simulink model "Lecture2_Exercise_Sim"  (R2023b)
settings: Solver=VariableStepAuto  StartTime=0.0  StopTime=5  RelTol=1e-3
values from neighbouring files (symbols this model uses):
  Bm = 5 * 10^(-3)    (= 0.005)    [Lab_Assignment_5XWB0.m]
  Jm = 16.9 * 10^(-3)    (= 0.0169)    [Lab_Assignment_5XWB0.m]
  Kb = 1.01    [Lab_Assignment_5XWB0.m]
  La = 10.8 * 10^(-3)    (= 0.0108)    [Lab_Assignment_5XWB0.m]
  Lf = 58.4    [Lab_Assignment_5XWB0.m]
  Ra = 1.93    [Lab_Assignment_5XWB0.m]
  Rf = 276    [Lab_Assignment_5XWB0.m]
  Tl = 5    [Lab_Assignment_5XWB0.m]
  Vfmax = 310    [Lab_Assignment_5XWB0.m]
settings Model: Creator=20210999  LastModifiedBy=20210999

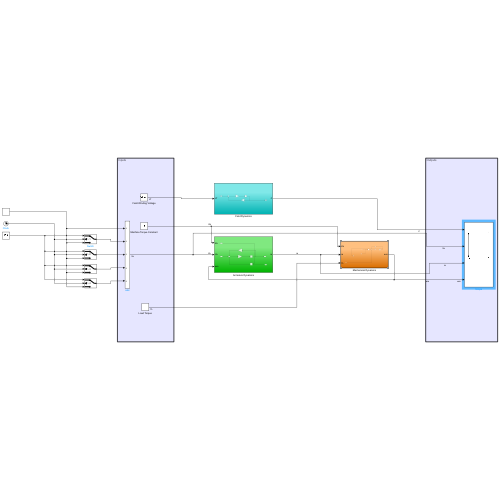
[thumbnail: Simulink's stored preview of the top-level diagram]
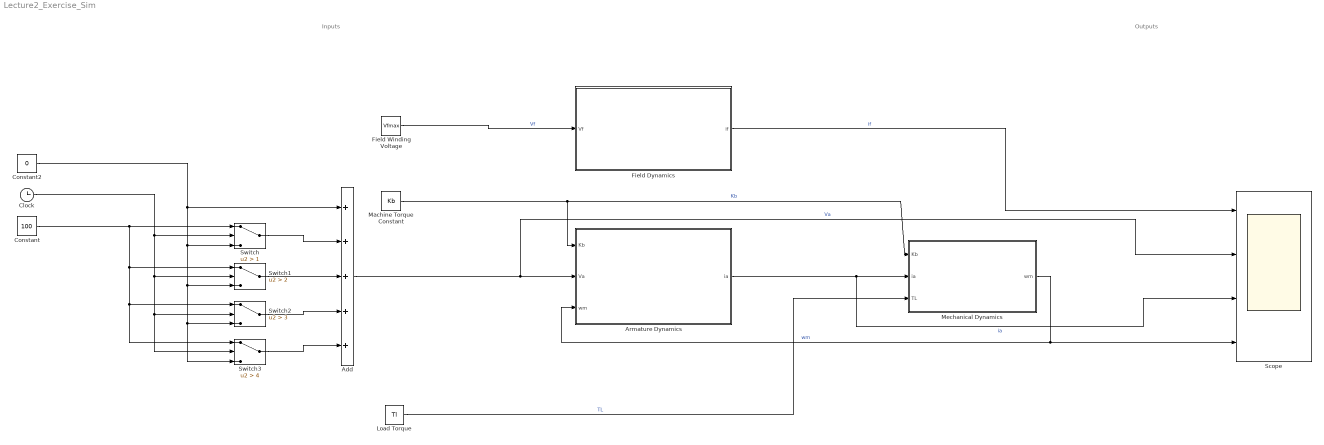
== system Lecture2_Exercise_Sim ==
  note: Inputs
  note: Outputs
  Add : Sum  Inputs=+++++
  Armature Dynamics : Subsystem
  Clock : Clock
      settings: Decimation=5
  Constant : Constant  Value=100
  Constant2 : Constant  Value=0
  Field Dynamics : Subsystem
  Field Winding Voltage : Constant  Value=Vfmax
  Load Torque : Constant  Value=Tl
  Machine Torque Constant : Constant  Value=Kb
  Mechanical Dynamics : Subsystem
  Scope : Scope  NumInputPorts=4
  Switch : Switch  Criteria=u2 > Threshold  Threshold=1  SaturateOnIntegerOverflow=off  InputSameDT=off
  Switch1 : Switch  Criteria=u2 > Threshold  Threshold=2  SaturateOnIntegerOverflow=off  InputSameDT=off
  Switch2 : Switch  Criteria=u2 > Threshold  Threshold=3  SaturateOnIntegerOverflow=off  InputSameDT=off
  Switch3 : Switch  Criteria=u2 > Threshold  Threshold=4  SaturateOnIntegerOverflow=off  InputSameDT=off
  wires:
  Field Winding Voltage/1 -> Field Dynamics/1(Vf)  "Vf"
  Machine Torque Constant/1 -> Armature Dynamics/1(Kb), Mechanical Dynamics/1(Kb)  "Kb"
  Armature Dynamics/1(ia) -> Scope/3, Mechanical Dynamics/2(ia)  "ia"
  Load Torque/1 -> Mechanical Dynamics/3(TL)  "TL"
  Mechanical Dynamics/1(wm) -> Scope/4, Armature Dynamics/3(wm)  "wm"
  Field Dynamics/1(if) -> Scope/1  "if"
  Clock/1 -> Switch3/2, Switch2/2, Switch1/2, Switch/2
  Constant2/1 -> Switch3/3, Switch2/3, Switch1/3, Switch/3, Add/1
  Switch/1 -> Add/2
  Switch1/1 -> Add/3
  Switch2/1 -> Add/4
  Switch3/1 -> Add/5
  Add/1 -> Scope/2, Armature Dynamics/2(Va)  "Va"
  Constant/1 -> Switch3/1, Switch2/1, Switch1/1, Switch/1

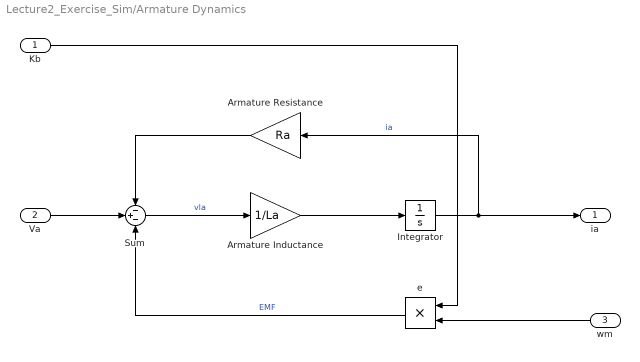
== system Lecture2_Exercise_Sim/Armature Dynamics ==
  Kb : Inport
  Va : Inport  Port=2
  wm : Inport  Port=3
  Armature Inductance : Gain  Gain=1/La
  Armature Resistance : Gain  Gain=Ra
  Integrator : Integrator
  Sum : Sum  Inputs=-+-
  e : Product
  ia : Outport
  wires:
  Integrator/1 -> ia/1, Armature Resistance/1  "ia"
  e/1 -> Sum/3  "EMF"
  Armature Inductance/1 -> Integrator/1
  Sum/1 -> Armature Inductance/1  "vla"
  Kb/1 -> e/1
  Va/1 -> Sum/2
  Armature Resistance/1 -> Sum/1
  wm/1 -> e/2

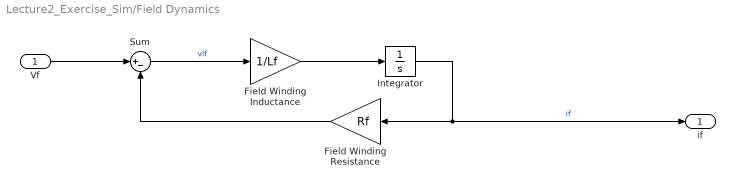
== system Lecture2_Exercise_Sim/Field Dynamics ==
  Vf : Inport
  Field Winding Inductance : Gain  Gain=1/Lf
  Field Winding Resistance : Gain  Gain=Rf
  Integrator : Integrator
  Sum : Sum  Inputs=|+-
  if : Outport
  wires:
  Field Winding Resistance/1 -> Sum/2
  Integrator/1 -> Field Winding Resistance/1, if/1  "if"
  Sum/1 -> Field Winding Inductance/1  "vlf"
  Vf/1 -> Sum/1
  Field Winding Inductance/1 -> Integrator/1

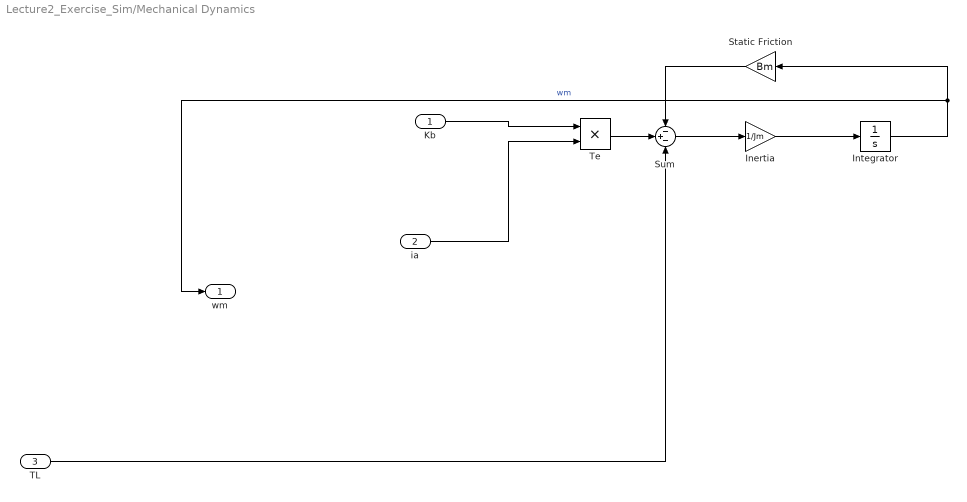
== system Lecture2_Exercise_Sim/Mechanical Dynamics ==
  Kb : Inport
  ia : Inport  Port=2
  TL : Inport  Port=3
  Inertia : Gain  Gain=1/Jm
  Integrator : Integrator
  Static Friction : Gain  Gain=Bm
  Sum : Sum  Inputs=-+-
  Te : Product
  wm : Outport
  wires:
  Kb/1 -> Te/1
  Te/1 -> Sum/2
  Static Friction/1 -> Sum/1
  Inertia/1 -> Integrator/1
  Integrator/1 -> wm/1, Static Friction/1  "wm"
  Sum/1 -> Inertia/1
  TL/1 -> Sum/3
  ia/1 -> Te/2
